simulink model "NEDnavV3"  (R2014a)
settings: Solver=FixedStepDiscrete  StartTime=0.0  StopTime=inf  FixedStep=0.1  RelTol=1e-3
libraries: simulink x1
settings Model: BufferReuse=off  Creator=wildcat  LastModifiedBy=wildcat
settings SolverCC: EnableConcurrentExecution=on
settings DataIOCC: SignalLoggingSaveFormat=ModelDataLogs
settings OptimizationCC: BlockReduction=off  OptimizeBlockIOStorage=off  BufferReuse=off  GlobalBufferReuse=off  ExpressionFolding=off  LocalBlockOutputs=off
settings DebuggingCC: UnderspecifiedInitializationDetection=Classic  MultiTaskDSMMsg=warning  StateNameClashWarn=warning
settings HardwareCC: ProdIntDivRoundTo=Zero  ProdEndianess=LittleEndian  ProdHWDeviceType=Generic->32-bit x86 compatible
settings RTWCC: SystemTargetFile=slrt.tlc  TemplateMakefile=slrt_default_tmf  Description=Simulink Real-Time  ProcessScript=slrt_make_rtw_hook  RTWCompilerOptimization=On
settings SimulinkRealTimeCC: GeneratePreprocessorConditionals=Disable all  EnableShiftOperators=on

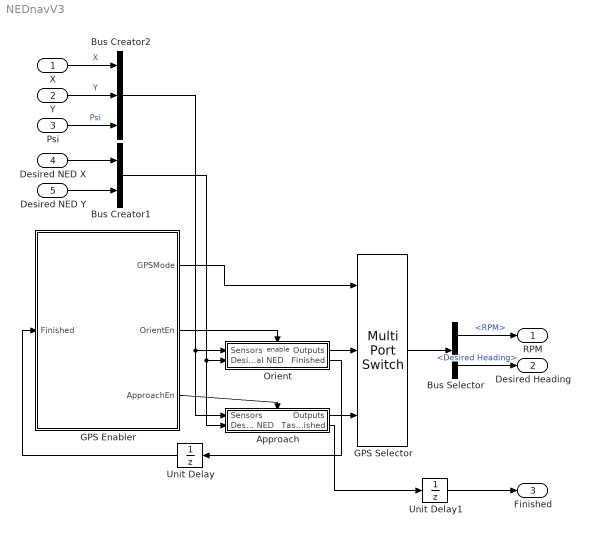
== system NEDnavV3 ==
  X : Inport
  Y : Inport  Port=2
  Psi : Inport  Port=3
  Desired NED X : Inport  Port=4
  Desired NED Y : Inport  Port=5
  Approach : Subsystem  TreatAsAtomicUnit=on
  Bus Creator1 : BusCreator  Inputs=2
  Bus Creator2 : BusCreator  Inputs=3
  Bus Selector : BusSelector  OutputSignals=RPM,Desired Heading
  GPS Enabler : MATLAB Function  TreatAsAtomicUnit=on
  GPS Selector : MultiPortSwitch  Inputs=2
  Orient : Subsystem  TreatAsAtomicUnit=on
  Unit Delay : UnitDelay  SampleTime=-1
  Unit Delay1 : UnitDelay  SampleTime=-1
  RPM : Outport
  Desired Heading : Outport  Port=2
  Finished : Outport  Port=3
  wires:
  Bus Creator2/1 -> Approach/1(Sensors), Orient/1(Sensors)
  GPS Enabler/2(OrientEn) -> Orient/Enable
  GPS Enabler/3(ApproachEn) -> Approach/Enable
  Orient/2(Finished) -> Unit Delay/1
  Orient/1(Outputs) -> GPS Selector/2
  Approach/1(Outputs) -> GPS Selector/3
  GPS Enabler/1(GPSMode) -> GPS Selector/1
  Unit Delay/1 -> GPS Enabler/1(Finished)
  GPS Selector/1 -> Bus Selector/1
  Approach/2(Task Finished) -> Unit Delay1/1
  Unit Delay1/1 -> Finished/1
  Bus Creator1/1 -> Approach/2(Desired Goal NED), Orient/2(Desired Goal NED)
  Psi/1 -> Bus Creator2/3  "Psi"
  Y/1 -> Bus Creator2/2  "Y"
  X/1 -> Bus Creator2/1  "X"
  Bus Selector/1 -> RPM/1  "<RPM>"
  Bus Selector/2 -> Desired Heading/1  "<Desired Heading>"
  Desired NED X/1 -> Bus Creator1/1
  Desired NED Y/1 -> Bus Creator1/2

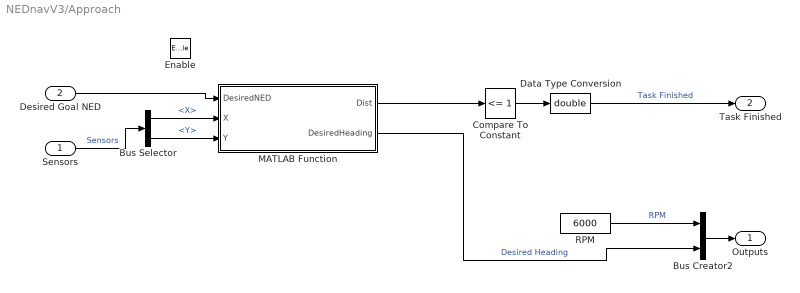
== system NEDnavV3/Approach ==
  Sensors : Inport
  Desired Goal NED : Inport  Port=2
  Enable : EnablePort
  Bus Creator2 : BusCreator  Inputs=2
  Bus Selector : BusSelector  OutputSignals=X,Y
  Compare To Constant : simulink/Logic and Bit Operations/Compare To Constant  relop=<=  const=1  OutDataTypeStr=boolean
  Data Type Conversion : DataTypeConversion  OutDataTypeStr=double
  MATLAB Function : MATLAB Function  TreatAsAtomicUnit=on
  RPM : Constant  Value=6000  SampleTime=-1
  Outputs : Outport
  Task Finished : Outport  Port=2
  wires:
  Sensors/1 -> Bus Selector/1  "Sensors"
  Bus Selector/1 -> MATLAB Function/2(X)  "<X>"
  Bus Selector/2 -> MATLAB Function/3(Y)  "<Y>"
  MATLAB Function/2(DesiredHeading) -> Bus Creator2/2  "Desired Heading"
  MATLAB Function/1(Dist) -> Compare To Constant/1
  Data Type Conversion/1 -> Task Finished/1  "Task Finished"
  Compare To Constant/1 -> Data Type Conversion/1
  Desired Goal NED/1 -> MATLAB Function/1(DesiredNED)
  RPM/1 -> Bus Creator2/1  "RPM"
  Bus Creator2/1 -> Outputs/1

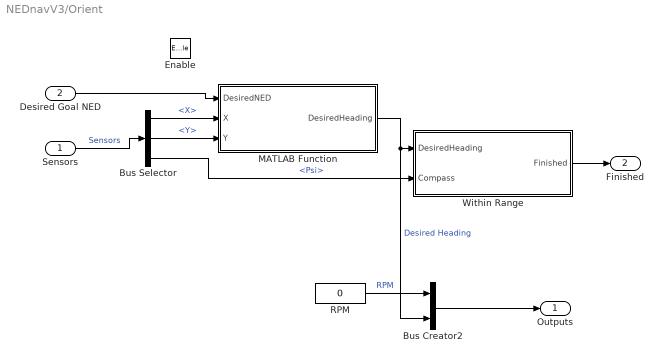
== system NEDnavV3/Orient ==
  Sensors : Inport
  Desired Goal NED : Inport  Port=2
  Enable : EnablePort
  Bus Creator2 : BusCreator  Inputs=2
  Bus Selector : BusSelector  OutputSignals=X,Y,Psi
  MATLAB Function : MATLAB Function  TreatAsAtomicUnit=on
  RPM : Constant  Value=0  SampleTime=-1
  Within Range : MATLAB Function  TreatAsAtomicUnit=on
  Outputs : Outport
  Finished : Outport  Port=2
  wires:
  Sensors/1 -> Bus Selector/1  "Sensors"
  Desired Goal NED/1 -> MATLAB Function/1(DesiredNED)
  Bus Selector/1 -> MATLAB Function/2(X)  "<X>"
  Bus Selector/2 -> MATLAB Function/3(Y)  "<Y>"
  MATLAB Function/1(DesiredHeading) -> Bus Creator2/2, Within Range/1(DesiredHeading)  "Desired Heading"
  Bus Selector/3 -> Within Range/2(Compass)  "<Psi>"
  Within Range/1(Finished) -> Finished/1
  RPM/1 -> Bus Creator2/1  "RPM"
  Bus Creator2/1 -> Outputs/1

== matlab function NEDnavV3/GPS Enabler ==
  data: Finished input; GPSMode output; OrientEn output; ApproachEn output
function [GPSMode, OrientEn, ApproachEn] = GPSEnable(Finished)

%Written by Anderson Lebbad on July 22, 2013
%Last Edited: July 27, 2013
%   Removed Termination Block

%This function enables GPS tasks. First the boat orients towards the
%target, then it approaches it.


%Parse Finished signal
OrientFinished = Finished(1);


%Initialize Enablers
OrientEn = 0;
ApproachEn = 0;


%Switches the enable signal based on which task is flagged as done.
if OrientFinished == 0
    OrientEn = 1;
    GPSMode = 1;
else
    ApproachEn = 1;
    GPSMode = 2;
end

== matlab function NEDnavV3/Approach/MATLAB Function ==
  data: Dist output; DesiredNED input; DesiredHeading output; X input; Y input
function [Dist, DesiredHeading] = HeadingDistNED(DesiredNED, X, Y)
%Written By Anderson Lebbad on June 7, 2015
%Last Edited by:

%This function determines a desired heading based off the current position
%and desired goal position in NED coordinates and distance to target

relX = DesiredNED(1) - X;
relY = DesiredNED(2) - Y;

DesiredHeading = atan2(relY, relX)*180/pi;
Dist = sqrt(relX.^2+relY.^2);

== matlab function NEDnavV3/Orient/MATLAB Function ==
  data: DesiredNED input; DesiredHeading output; X input; Y input
function DesiredHeading = HeadingNED(DesiredNED, X, Y)
%Written By Anderson Lebbad on June 7, 2015
%Last Edited by:

%This function determines a desired heading based off the current position
%and desired goal position in NED coordinates

relX = DesiredNED(1) - X;
relY = DesiredNED(2) - Y;

DesiredHeading = atan2(relY, relX)*180/pi;

== matlab function NEDnavV3/Orient/Within Range ==
  data: DesiredHeading input; Finished output; Compass input
function Finished = OrientLocked(DesiredHeading, Compass)

%Written by Anderson Lebbad on July 22, 2013
%Last Edited:

%This function checks to see if the target heading has been reached and 
%sends a finished signal when it has.
persistent counter
if isempty(counter)
    counter = 0;
end

HeadingDiff = DesiredHeading - Compass;

%Sets the range for the difference angle to be -180 to +180
if HeadingDiff > 180
    HeadingDiff = HeadingDiff - 360;
elseif HeadingDiff < -180
    HeadingDiff = HeadingDiff + 360;
end

%If the Heading is within 3 degrees, the angle is close enough to send a
%finished signal
if abs(HeadingDiff) < 15
    counter = counter + 1;
    if counter >= 10;
        Finished = 1;
    else
        Finished = 0;
    end
else
    counter = 0;
    Finished = 0;
end
